simulink model "product_matrix_test"  (Simulink 8.4)
settings: Solver=ode45  StartTime=0.0  StopTime=10.0  RelTol=1e-3
settings Model: Creator=arnaud  LastModifiedBy=arnaud
settings DataIOCC: SaveFormat=Structure

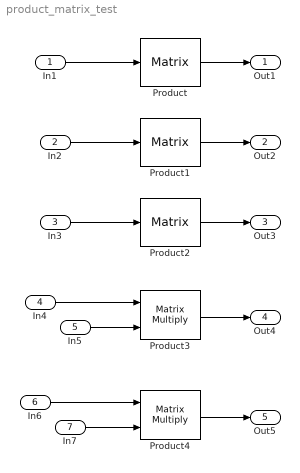
== system product_matrix_test ==
  In1 : Inport
  In2 : Inport  Port=2  PortDimensions=3
  In3 : Inport  Port=3  PortDimensions=[2 3]
  In4 : Inport  Port=4  PortDimensions=[2 3]
  In5 : Inport  Port=5  PortDimensions=[3 3]
  In6 : Inport  Port=6  PortDimensions=[1 2]
  In7 : Inport  Port=7  PortDimensions=[2 1]
  Product : Product  Inputs=1  Multiplication=Matrix(*)  RndMeth=Zero
  Product1 : Product  Inputs=1  Multiplication=Matrix(*)  RndMeth=Zero
  Product2 : Product  Inputs=1  Multiplication=Matrix(*)  RndMeth=Zero
  Product3 : Product  Inputs=**  Multiplication=Matrix(*)  RndMeth=Zero
  Product4 : Product  Inputs=**  Multiplication=Matrix(*)  RndMeth=Zero
  Out1 : Outport
  Out2 : Outport  Port=2
  Out3 : Outport  Port=3
  Out4 : Outport  Port=4
  Out5 : Outport  Port=5
  wires:
  In1/1 -> Product/1
  Product/1 -> Out1/1
  In2/1 -> Product1/1
  Product1/1 -> Out2/1
  In3/1 -> Product2/1
  Product2/1 -> Out3/1
  In4/1 -> Product3/1
  Product3/1 -> Out4/1
  In5/1 -> Product3/2
  In6/1 -> Product4/1
  Product4/1 -> Out5/1
  In7/1 -> Product4/2
